simulink model "L1_4"  (Simulink 7.9)
settings: Solver=ode45  StartTime=0.0  StopTime=0.31  RelTol=1e-3
libraries: simulink x1
settings Model: Creator=Павло  LastModifiedBy=Павло

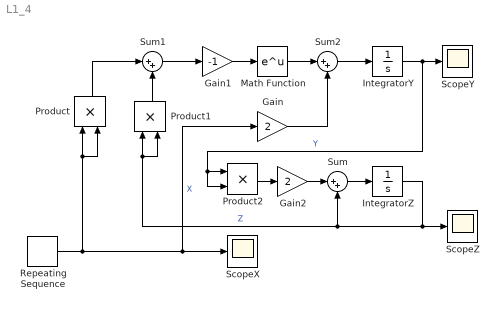
== system L1_4 ==
  Gain : Gain  Gain=2
  Gain1 : Gain  Gain=-1
  Gain2 : Gain  Gain=2
  IntegratorY : Integrator  InitialCondition=0.5
  IntegratorZ : Integrator  InitialCondition=1
  Math Function : Math  SaturateOnIntegerOverflow=on
  Product : Product  RndMeth=Zero
  Product1 : Product  RndMeth=Zero
  Product2 : Product  RndMeth=Zero
  Repeating Sequence : simulink/Sources/Repeating Sequence  rep_seq_t=[0 4]  rep_seq_y=[0 4]
  ScopeX : Scope
      settings: TickLabels=on  TimeRange=0.9379378758757522  YMin=0.2922020202020199  YMax=0.54820202020202  SaveName=ScopeData2
  ScopeY : Scope
  ScopeZ : Scope
      settings: TickLabels=on  TimeRange=0.9379378758757522  YMin=0.2922020202020199  YMax=0.54820202020202
  Sum : Sum  Inputs=|++
  Sum1 : Sum  Inputs=|++
  Sum2 : Sum  Inputs=|++
  wires:
  IntegratorZ/1 -> ScopeZ/1, Product1/1, Product1/2, Sum/2  "Z"
  IntegratorY/1 -> ScopeY/1, Product2/2, Product2/1  "Y"
  Sum2/1 -> IntegratorY/1
  Repeating Sequence/1 -> Product/1, Product/2, ScopeX/1, Gain/1  "X"
  Math Function/1 -> Sum2/1
  Sum/1 -> IntegratorZ/1
  Product/1 -> Sum1/1
  Product1/1 -> Sum1/2
  Gain1/1 -> Math Function/1
  Sum1/1 -> Gain1/1
  Gain2/1 -> Sum/1
  Product2/1 -> Gain2/1
  Gain/1 -> Sum2/2
